simulink model "sim12ex4"  (Simulink 2.09)
settings: Solver=ode45  StartTime=0.0  StopTime=25  MaxStep=.1  RelTol=1e-3  AbsTol=1e-3
settings Model: SaveTime=off  SaveOutput=off  ConsistencyChecking=off  RTWTemplateMakefile=grt_vc.tmf

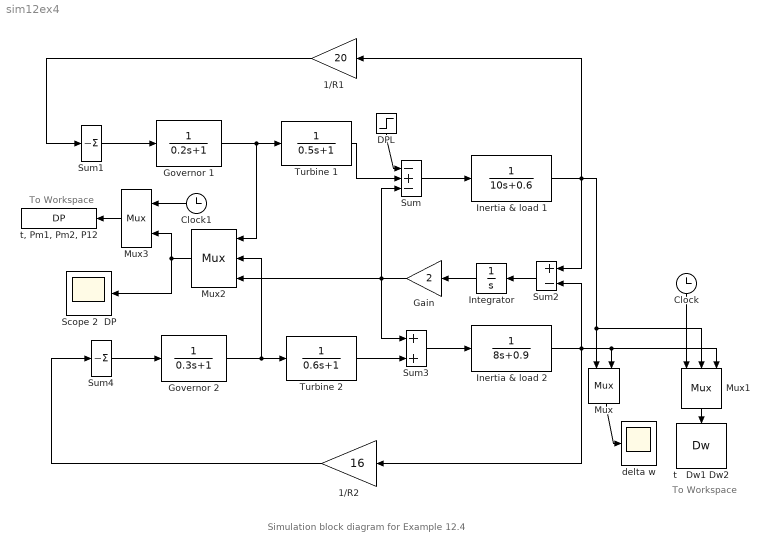
== system sim12ex4 ==
  note: To Workspace
  note: To Workspace
  note: Simulation block diagram for Example 12.4
  "   Governor 2" : TransferFcn  Numerator=[1]  Denominator="[0.3   1]"
  " Governor 1" : TransferFcn  Numerator=[1]  Denominator="[0.2   1]"
  " Turbine 1" : TransferFcn  Numerator=[1]  Denominator="[0.5  1]"
  " delta w  " : Scope
      settings: TickLabels=on  TimeRange=auto  YMin=-5  YMax=5  SaveToWorkspace=off  SaveName=ScopeData
  1/R1 : Gain  Orientation=left  Gain=20
  1/R2 : Gain  Orientation=left  Gain=16
  Clock : Clock
      settings: Orientation=down
  Clock1 : Clock
  "DPL " : Step  Orientation=down  Time=100  Before=0.1875  After=.1875
  Gain : Gain  Orientation=left  Gain=2
  "Inertia & load 1 " : TransferFcn  Numerator=[1]  Denominator="[10  0.6]"
  Inertia & load 2 : TransferFcn  Numerator=[1]  Denominator="[8  0.9]"
  Integrator : Integrator  Orientation=left  ExternalReset=none  InitialConditionSource=internal  InitialCondition=0  LimitOutput=off  UpperSaturationLimit=inf  LowerSaturationLimit=-inf  ShowSaturationPort=off  ShowStatePort=off  AbsoluteTolerance=auto
  Mux : Mux  Orientation=down  Inputs=2
  Mux1 : Mux  Orientation=down  Inputs=3
  Mux2 : Mux  Orientation=left  Inputs=3
  Mux3 : Mux  Orientation=left  Inputs=2
  Scope 2  DP : Scope
      settings: TickLabels=on  TimeRange=auto  YMin=-5  YMax=5  SaveToWorkspace=off  SaveName=ScopeData
  Sum : Sum  Inputs=-+-
  Sum1 : Sum  Inputs=-
  Sum2 : Sum  Orientation=left  Inputs=+-
  Sum3 : Sum  Inputs=++
  Sum4 : Sum  Inputs=-
  Turbine 2 : TransferFcn  Numerator=[1]  Denominator="[0.6  1]"
  t   Dw1 Dw2 : ToWorkspace  VariableName=Dw  SampleTime=0
      settings: Orientation=down  Buffer=1000
  "t, Pm1, Pm2, P12" : ToWorkspace  VariableName=DP  SampleTime=0
      settings: Buffer=1000
  wires:
  Gain/1 -> Sum3/1, Sum/3, Mux2/3
  Clock/1 -> Mux1/1
  Mux1/1 -> t   Dw1 Dw2/1
  "Inertia & load 1 "/1 -> Mux1/2, Mux/1, Sum2/1, 1/R1/1
  Inertia & load 2/1 -> Mux/2, Mux1/3, Sum2/2, 1/R2/1
  1/R2/1 -> Sum4/1
  Turbine 2/1 -> Sum3/2
  Sum4/1 -> "   Governor 2"/1
  Sum3/1 -> Inertia & load 2/1
  Integrator/1 -> Gain/1
  Sum2/1 -> Integrator/1
  1/R1/1 -> Sum1/1
  "DPL "/1 -> Sum/1
  Sum1/1 -> " Governor 1"/1
  Sum/1 -> "Inertia & load 1 "/1
  " Turbine 1"/1 -> Sum/2
  Mux/1 -> " delta w  "/1
  " Governor 1"/1 -> " Turbine 1"/1, Mux2/1
  "   Governor 2"/1 -> Turbine 2/1, Mux2/2
  Clock1/1 -> Mux3/1
  Mux3/1 -> "t, Pm1, Pm2, P12"/1
  Mux2/1 -> Scope 2  DP/1, Mux3/2
